simulink model "SIM_PEM_stack"  (R2020b)
settings: Solver=VariableStepAuto  StartTime=0.0  StopTime=60e3  RelTol=1e-3
undefined symbols (not defined in the file or in its folder): FC, FuelCellLoadFcn, gcbh, sps_rtmsupport
libraries: powerlib x106, simulink x22, spsFuelCellModel x21, dspswit3 x1, mylib x1
(part 2 of 3)

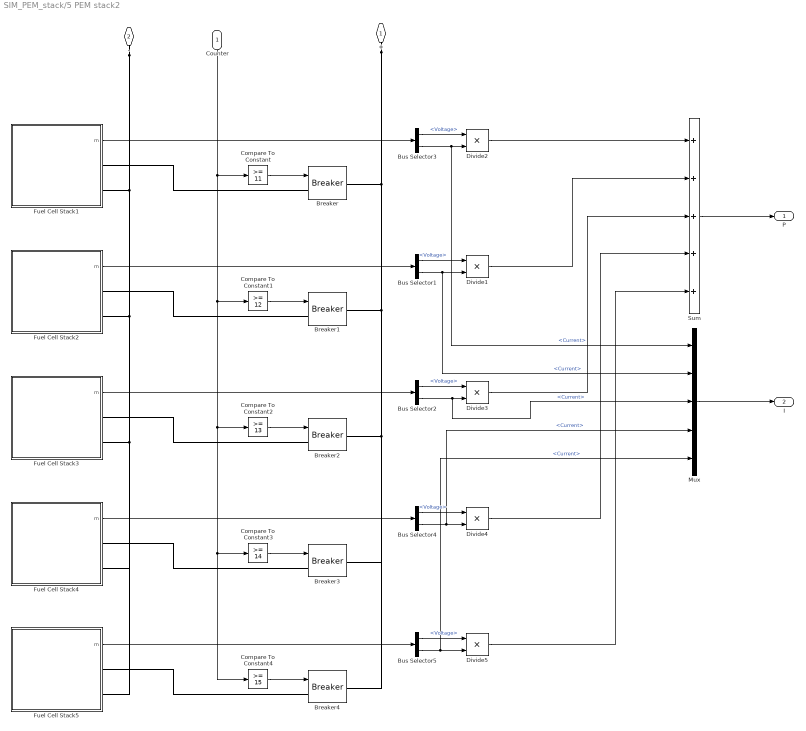
== system SIM_PEM_stack/5 PEM stack2 ==
  Counter : Inport
  Breaker{,1..4} (5 alike) : powerlib/Elements/Breaker  InitialState=0  SwitchingTimes="[1/60  5/60]"  External=on  BreakerResistance=0.01  SnubberResistance=1e6  SnubberCapacitance=inf  Measurements=None  MoreParameters=on  NoBreakLoop=off
  Bus Selector{1..5} (5 alike) : BusSelector  OutputSignals=Voltage,Current
  Compare To Constant : simulink/Logic and Bit Operations/Compare To Constant  relop=>=  const=11  OutDataTypeStr=boolean
  Compare To Constant1 : simulink/Logic and Bit Operations/Compare To Constant  relop=>=  const=12  OutDataTypeStr=boolean
  Compare To Constant2 : simulink/Logic and Bit Operations/Compare To Constant  relop=>=  const=13  OutDataTypeStr=boolean
  Compare To Constant3 : simulink/Logic and Bit Operations/Compare To Constant  relop=>=  const=14  OutDataTypeStr=boolean
  Compare To Constant4 : simulink/Logic and Bit Operations/Compare To Constant  relop=>=  const=15  OutDataTypeStr=boolean
  Divide{1..5} (5 alike) : Product  Inputs=**
  Fuel Cell Stack1 : Subsystem  AncestorBlock=electricdrivelib/Extra Sources/Fuel Cell Stack  DialogController=POWERSYS.PowerSysDialog  LoadFcn=sps_rtmsupport('LoadFcn',gcbh);FuelCellLoadFcn(gcb)  StartFcn=sps_rtmsupport('StartFcn',gcbh);  StopFcn=sps_rtmsupport('StopFcn',gcbh);  mask(Fuel Cell Stack){PresetModel=No (User-Defined), FcType=Proton Exchange Membrane (PEM), Detailed=Detailed, Eoc=[93.2,88], NomVI=[160,65.5], EndVI=[230,58.6], Nc=96, n=54, TOp=65, AirFr=510, SuppPress=[1.26,1], Comp=[99.95,21,1], SignX=off, SignY=off, FlowRateH2=off, FlowRateAir=off, SystemTemp=off, SystemPH2=off, SystemPAir=off, FCDyn=on, FC_tau=1, Peak_O2=80, V_Under=10}
      mask prompts: PresetModel "Preset model:"; FcType "Fuel Cell type:"; Detailed "Model detail Level:"; Eoc "Voltage at 0A and 1A [V_0(V), V_1(V)]"; NomVI "Nominal operating point [Inom(A), Vnom(V)]"; EndVI "Maximum operating point [Iend(A), Vend(V)]"; Nc "Number of cells"; n "Nominal stack efficiency (%)"; TOp "Operating temperature (Celsius)"; AirFr "Nominal Air flow rate (lpm)"; SuppPress "Nominal supply pressure [Fuel (bar), Air (bar)]"; Comp "Nominal composition (%) [H2 O2 H2O(Air)]"; SignX "Fuel  composition [x_H2(%)]"; SignY "Oxidant composition [y_O2(%)]"; FlowRateH2 "Fuel flow rate [FuelFr(lpm)]"; FlowRateAir "Air flow rate [AirFr(lpm)]"; SystemTemp "System Temperature [T(Kelvin)]"; SystemPH2 "Fuel supply pressure [Pfuel(bar)]"; SystemPAir "Air supply pressure [PAir(bar)]"; FCDyn "Specify Fuel Cell Dynamics?"; FC_tau "Fuel Cell response time (sec)"; Peak_O2 "Peak O2 utilization (%)"; V_Under "Voltage undershoot (V) @ peak O2 utilization"
      mask help:
      | Implements a generic hydrogen fuel cell model which allows the simulation for the following types of cells:
      | - Proton Exchange Membrane Fuel Cell (PEMFC)
      | - Solid Oxide Fuel Cell (SOFC)
      | - Alkaline Fuel Cell (AFC)
      mask init: same as SIM_PEM_stack/Fuel Cell Stack
      settings: CopyFcn=sps_rtmsupport('CopyFcn',gcbh);  DeleteFcn=sps_rtmsupport('DeleteFcn',gcbh);  UndoDeleteFcn=sps_rtmsupport('UndoDeleteFcn',gcbh);  ModelCloseFcn=sps_rtmsupport('ModelCloseFcn',gcbh);  PreSaveFcn=sps_rtmsupport('PreSaveFcn',gcbh);  PostSaveFcn=sps_rtmsupport('PostSaveFcn',gcbh);  NameChangeFcn=sps_rtmsupport('NameChangeFcn',gcbh);  PreCopyFcn=sps_rtmsupport('PreCopyFcn',gcbh);  OpenFcn=sps_rtmsupport('OpenFcn',gcbh, [1 2 3 13 14 15 16 17 18 19 20]);  CloseFcn=sps_rtmsupport('CloseFcn',gcbh);  PreDeleteFcn=sps_rtmsupport('PreDeleteFcn',gcbh);
      mask Help: helpview(psbhelp)
      mask TypeOptions PresetModel: No (User-Defined) | PEMFC - 1.26 kW - 24 Vdc | PEMFC - 6 kW - 45 Vdc | PEMFC - 50 kW - 625 Vdc | AFC - 2.4 kW - 48 Vdc | SOFC - 3 kW - 100 Vdc | SOFC - 25 kW - 630 Vdc
      mask Callback PresetModel: FuelCellCback(gcb,'Preset')
      mask TypeOptions Detailed: Simplified | Detailed
      mask Callback Detailed: FuelCellCback(gcb,'Visibilities')
      mask Callback FlowRateAir: FuelCellCback(gcb,'Visibilities')
      mask Callback FCDyn: FuelCellCback(gcb,'Visibilities')
      mask DialogControl ParameterTabVar0 Prompt: Parameters
      mask DialogControl plot_graph Prompt: Plot V_I characteristic
      mask DialogControl plot_graph Callback: FuelCellCback(gcb,'PlotGraph');
      mask DialogControl ViewParam Prompt: View Cell parameters
      mask DialogControl ViewParam Callback: FuelCellCback(gcb,'ViewParam');
      mask DialogControl ParameterTabVar01 Prompt: Signal variation
      mask DialogControl ParameterTabVar012 Prompt: Fuel Cell Dynamics
      mask Display: image(imread('power_fuelcell.png'));
  Fuel Cell Stack2 : Subsystem  AncestorBlock=electricdrivelib/Extra Sources/Fuel Cell Stack  DialogController=POWERSYS.PowerSysDialog  LoadFcn=sps_rtmsupport('LoadFcn',gcbh);FuelCellLoadFcn(gcb)  StartFcn=sps_rtmsupport('StartFcn',gcbh);  StopFcn=sps_rtmsupport('StopFcn',gcbh);  mask(Fuel Cell Stack){PresetModel=No (User-Defined), FcType=Proton Exchange Membrane (PEM), Detailed=Detailed, Eoc=[93.2,88], NomVI=[160,65.5], EndVI=[230,58.6], Nc=96, n=54, TOp=65, AirFr=510, SuppPress=[1.26,1], Comp=[99.95,21,1], SignX=off, SignY=off, FlowRateH2=off, FlowRateAir=off, SystemTemp=off, SystemPH2=off, SystemPAir=off, FCDyn=on, FC_tau=1, Peak_O2=80, V_Under=10}
      mask prompts: PresetModel "Preset model:"; FcType "Fuel Cell type:"; Detailed "Model detail Level:"; Eoc "Voltage at 0A and 1A [V_0(V), V_1(V)]"; NomVI "Nominal operating point [Inom(A), Vnom(V)]"; EndVI "Maximum operating point [Iend(A), Vend(V)]"; Nc "Number of cells"; n "Nominal stack efficiency (%)"; TOp "Operating temperature (Celsius)"; AirFr "Nominal Air flow rate (lpm)"; SuppPress "Nominal supply pressure [Fuel (bar), Air (bar)]"; Comp "Nominal composition (%) [H2 O2 H2O(Air)]"; SignX "Fuel  composition [x_H2(%)]"; SignY "Oxidant composition [y_O2(%)]"; FlowRateH2 "Fuel flow rate [FuelFr(lpm)]"; FlowRateAir "Air flow rate [AirFr(lpm)]"; SystemTemp "System Temperature [T(Kelvin)]"; SystemPH2 "Fuel supply pressure [Pfuel(bar)]"; SystemPAir "Air supply pressure [PAir(bar)]"; FCDyn "Specify Fuel Cell Dynamics?"; FC_tau "Fuel Cell response time (sec)"; Peak_O2 "Peak O2 utilization (%)"; V_Under "Voltage undershoot (V) @ peak O2 utilization"
      mask help:
      | Implements a generic hydrogen fuel cell model which allows the simulation for the following types of cells:
      | - Proton Exchange Membrane Fuel Cell (PEMFC)
      | - Solid Oxide Fuel Cell (SOFC)
      | - Alkaline Fuel Cell (AFC)
      mask init: same as SIM_PEM_stack/Fuel Cell Stack
      settings: CopyFcn=sps_rtmsupport('CopyFcn',gcbh);  DeleteFcn=sps_rtmsupport('DeleteFcn',gcbh);  UndoDeleteFcn=sps_rtmsupport('UndoDeleteFcn',gcbh);  ModelCloseFcn=sps_rtmsupport('ModelCloseFcn',gcbh);  PreSaveFcn=sps_rtmsupport('PreSaveFcn',gcbh);  PostSaveFcn=sps_rtmsupport('PostSaveFcn',gcbh);  NameChangeFcn=sps_rtmsupport('NameChangeFcn',gcbh);  PreCopyFcn=sps_rtmsupport('PreCopyFcn',gcbh);  OpenFcn=sps_rtmsupport('OpenFcn',gcbh, [1 2 3 13 14 15 16 17 18 19 20]);  CloseFcn=sps_rtmsupport('CloseFcn',gcbh);  PreDeleteFcn=sps_rtmsupport('PreDeleteFcn',gcbh);
      mask Help: helpview(psbhelp)
      mask TypeOptions PresetModel: No (User-Defined) | PEMFC - 1.26 kW - 24 Vdc | PEMFC - 6 kW - 45 Vdc | PEMFC - 50 kW - 625 Vdc | AFC - 2.4 kW - 48 Vdc | SOFC - 3 kW - 100 Vdc | SOFC - 25 kW - 630 Vdc
      mask Callback PresetModel: FuelCellCback(gcb,'Preset')
      mask TypeOptions Detailed: Simplified | Detailed
      mask Callback Detailed: FuelCellCback(gcb,'Visibilities')
      mask Callback FlowRateAir: FuelCellCback(gcb,'Visibilities')
      mask Callback FCDyn: FuelCellCback(gcb,'Visibilities')
      mask DialogControl ParameterTabVar0 Prompt: Parameters
      mask DialogControl plot_graph Prompt: Plot V_I characteristic
      mask DialogControl plot_graph Callback: FuelCellCback(gcb,'PlotGraph');
      mask DialogControl ViewParam Prompt: View Cell parameters
      mask DialogControl ViewParam Callback: FuelCellCback(gcb,'ViewParam');
      mask DialogControl ParameterTabVar01 Prompt: Signal variation
      mask DialogControl ParameterTabVar012 Prompt: Fuel Cell Dynamics
      mask Display: image(imread('power_fuelcell.png'));
  Fuel Cell Stack3 : Subsystem  AncestorBlock=electricdrivelib/Extra Sources/Fuel Cell Stack  DialogController=POWERSYS.PowerSysDialog  LoadFcn=sps_rtmsupport('LoadFcn',gcbh);FuelCellLoadFcn(gcb)  StartFcn=sps_rtmsupport('StartFcn',gcbh);  StopFcn=sps_rtmsupport('StopFcn',gcbh);  mask(Fuel Cell Stack){PresetModel=No (User-Defined), FcType=Proton Exchange Membrane (PEM), Detailed=Detailed, Eoc=[93.2,88], NomVI=[160,65.5], EndVI=[230,58.6], Nc=96, n=54, TOp=65, AirFr=510, SuppPress=[1.26,1], Comp=[99.95,21,1], SignX=off, SignY=off, FlowRateH2=off, FlowRateAir=off, SystemTemp=off, SystemPH2=off, SystemPAir=off, FCDyn=on, FC_tau=1, Peak_O2=80, V_Under=10}
      mask prompts: PresetModel "Preset model:"; FcType "Fuel Cell type:"; Detailed "Model detail Level:"; Eoc "Voltage at 0A and 1A [V_0(V), V_1(V)]"; NomVI "Nominal operating point [Inom(A), Vnom(V)]"; EndVI "Maximum operating point [Iend(A), Vend(V)]"; Nc "Number of cells"; n "Nominal stack efficiency (%)"; TOp "Operating temperature (Celsius)"; AirFr "Nominal Air flow rate (lpm)"; SuppPress "Nominal supply pressure [Fuel (bar), Air (bar)]"; Comp "Nominal composition (%) [H2 O2 H2O(Air)]"; SignX "Fuel  composition [x_H2(%)]"; SignY "Oxidant composition [y_O2(%)]"; FlowRateH2 "Fuel flow rate [FuelFr(lpm)]"; FlowRateAir "Air flow rate [AirFr(lpm)]"; SystemTemp "System Temperature [T(Kelvin)]"; SystemPH2 "Fuel supply pressure [Pfuel(bar)]"; SystemPAir "Air supply pressure [PAir(bar)]"; FCDyn "Specify Fuel Cell Dynamics?"; FC_tau "Fuel Cell response time (sec)"; Peak_O2 "Peak O2 utilization (%)"; V_Under "Voltage undershoot (V) @ peak O2 utilization"
      mask help:
      | Implements a generic hydrogen fuel cell model which allows the simulation for the following types of cells:
      | - Proton Exchange Membrane Fuel Cell (PEMFC)
      | - Solid Oxide Fuel Cell (SOFC)
      | - Alkaline Fuel Cell (AFC)
      mask init: same as SIM_PEM_stack/Fuel Cell Stack
      settings: CopyFcn=sps_rtmsupport('CopyFcn',gcbh);  DeleteFcn=sps_rtmsupport('DeleteFcn',gcbh);  UndoDeleteFcn=sps_rtmsupport('UndoDeleteFcn',gcbh);  ModelCloseFcn=sps_rtmsupport('ModelCloseFcn',gcbh);  PreSaveFcn=sps_rtmsupport('PreSaveFcn',gcbh);  PostSaveFcn=sps_rtmsupport('PostSaveFcn',gcbh);  NameChangeFcn=sps_rtmsupport('NameChangeFcn',gcbh);  PreCopyFcn=sps_rtmsupport('PreCopyFcn',gcbh);  OpenFcn=sps_rtmsupport('OpenFcn',gcbh, [1 2 3 13 14 15 16 17 18 19 20]);  CloseFcn=sps_rtmsupport('CloseFcn',gcbh);  PreDeleteFcn=sps_rtmsupport('PreDeleteFcn',gcbh);
      mask Help: helpview(psbhelp)
      mask TypeOptions PresetModel: No (User-Defined) | PEMFC - 1.26 kW - 24 Vdc | PEMFC - 6 kW - 45 Vdc | PEMFC - 50 kW - 625 Vdc | AFC - 2.4 kW - 48 Vdc | SOFC - 3 kW - 100 Vdc | SOFC - 25 kW - 630 Vdc
      mask Callback PresetModel: FuelCellCback(gcb,'Preset')
      mask TypeOptions Detailed: Simplified | Detailed
      mask Callback Detailed: FuelCellCback(gcb,'Visibilities')
      mask Callback FlowRateAir: FuelCellCback(gcb,'Visibilities')
      mask Callback FCDyn: FuelCellCback(gcb,'Visibilities')
      mask DialogControl ParameterTabVar0 Prompt: Parameters
      mask DialogControl plot_graph Prompt: Plot V_I characteristic
      mask DialogControl plot_graph Callback: FuelCellCback(gcb,'PlotGraph');
      mask DialogControl ViewParam Prompt: View Cell parameters
      mask DialogControl ViewParam Callback: FuelCellCback(gcb,'ViewParam');
      mask DialogControl ParameterTabVar01 Prompt: Signal variation
      mask DialogControl ParameterTabVar012 Prompt: Fuel Cell Dynamics
      mask Display: image(imread('power_fuelcell.png'));
  Fuel Cell Stack4 : Subsystem  AncestorBlock=electricdrivelib/Extra Sources/Fuel Cell Stack  DialogController=POWERSYS.PowerSysDialog  LoadFcn=sps_rtmsupport('LoadFcn',gcbh);FuelCellLoadFcn(gcb)  StartFcn=sps_rtmsupport('StartFcn',gcbh);  StopFcn=sps_rtmsupport('StopFcn',gcbh);  mask(Fuel Cell Stack){PresetModel=No (User-Defined), FcType=Proton Exchange Membrane (PEM), Detailed=Detailed, Eoc=[93.2,88], NomVI=[160,65.5], EndVI=[230,58.6], Nc=96, n=54, TOp=65, AirFr=510, SuppPress=[1.26,1], Comp=[99.95,21,1], SignX=off, SignY=off, FlowRateH2=off, FlowRateAir=off, SystemTemp=off, SystemPH2=off, SystemPAir=off, FCDyn=on, FC_tau=1, Peak_O2=80, V_Under=10}
      mask prompts: PresetModel "Preset model:"; FcType "Fuel Cell type:"; Detailed "Model detail Level:"; Eoc "Voltage at 0A and 1A [V_0(V), V_1(V)]"; NomVI "Nominal operating point [Inom(A), Vnom(V)]"; EndVI "Maximum operating point [Iend(A), Vend(V)]"; Nc "Number of cells"; n "Nominal stack efficiency (%)"; TOp "Operating temperature (Celsius)"; AirFr "Nominal Air flow rate (lpm)"; SuppPress "Nominal supply pressure [Fuel (bar), Air (bar)]"; Comp "Nominal composition (%) [H2 O2 H2O(Air)]"; SignX "Fuel  composition [x_H2(%)]"; SignY "Oxidant composition [y_O2(%)]"; FlowRateH2 "Fuel flow rate [FuelFr(lpm)]"; FlowRateAir "Air flow rate [AirFr(lpm)]"; SystemTemp "System Temperature [T(Kelvin)]"; SystemPH2 "Fuel supply pressure [Pfuel(bar)]"; SystemPAir "Air supply pressure [PAir(bar)]"; FCDyn "Specify Fuel Cell Dynamics?"; FC_tau "Fuel Cell response time (sec)"; Peak_O2 "Peak O2 utilization (%)"; V_Under "Voltage undershoot (V) @ peak O2 utilization"
      mask help:
      | Implements a generic hydrogen fuel cell model which allows the simulation for the following types of cells:
      | - Proton Exchange Membrane Fuel Cell (PEMFC)
      | - Solid Oxide Fuel Cell (SOFC)
      | - Alkaline Fuel Cell (AFC)
      mask init: same as SIM_PEM_stack/Fuel Cell Stack
      settings: CopyFcn=sps_rtmsupport('CopyFcn',gcbh);  DeleteFcn=sps_rtmsupport('DeleteFcn',gcbh);  UndoDeleteFcn=sps_rtmsupport('UndoDeleteFcn',gcbh);  ModelCloseFcn=sps_rtmsupport('ModelCloseFcn',gcbh);  PreSaveFcn=sps_rtmsupport('PreSaveFcn',gcbh);  PostSaveFcn=sps_rtmsupport('PostSaveFcn',gcbh);  NameChangeFcn=sps_rtmsupport('NameChangeFcn',gcbh);  PreCopyFcn=sps_rtmsupport('PreCopyFcn',gcbh);  OpenFcn=sps_rtmsupport('OpenFcn',gcbh, [1 2 3 13 14 15 16 17 18 19 20]);  CloseFcn=sps_rtmsupport('CloseFcn',gcbh);  PreDeleteFcn=sps_rtmsupport('PreDeleteFcn',gcbh);
      mask Help: helpview(psbhelp)
      mask TypeOptions PresetModel: No (User-Defined) | PEMFC - 1.26 kW - 24 Vdc | PEMFC - 6 kW - 45 Vdc | PEMFC - 50 kW - 625 Vdc | AFC - 2.4 kW - 48 Vdc | SOFC - 3 kW - 100 Vdc | SOFC - 25 kW - 630 Vdc
      mask Callback PresetModel: FuelCellCback(gcb,'Preset')
      mask TypeOptions Detailed: Simplified | Detailed
      mask Callback Detailed: FuelCellCback(gcb,'Visibilities')
      mask Callback FlowRateAir: FuelCellCback(gcb,'Visibilities')
      mask Callback FCDyn: FuelCellCback(gcb,'Visibilities')
      mask DialogControl ParameterTabVar0 Prompt: Parameters
      mask DialogControl plot_graph Prompt: Plot V_I characteristic
      mask DialogControl plot_graph Callback: FuelCellCback(gcb,'PlotGraph');
      mask DialogControl ViewParam Prompt: View Cell parameters
      mask DialogControl ViewParam Callback: FuelCellCback(gcb,'ViewParam');
      mask DialogControl ParameterTabVar01 Prompt: Signal variation
      mask DialogControl ParameterTabVar012 Prompt: Fuel Cell Dynamics
      mask Display: image(imread('power_fuelcell.png'));
  Fuel Cell Stack5 : Subsystem  AncestorBlock=electricdrivelib/Extra Sources/Fuel Cell Stack  DialogController=POWERSYS.PowerSysDialog  LoadFcn=sps_rtmsupport('LoadFcn',gcbh);FuelCellLoadFcn(gcb)  StartFcn=sps_rtmsupport('StartFcn',gcbh);  StopFcn=sps_rtmsupport('StopFcn',gcbh);  mask(Fuel Cell Stack){PresetModel=No (User-Defined), FcType=Proton Exchange Membrane (PEM), Detailed=Detailed, Eoc=[93.2,88], NomVI=[160,65.5], EndVI=[230,58.6], Nc=96, n=54, TOp=65, AirFr=510, SuppPress=[1.26,1], Comp=[99.95,21,1], SignX=off, SignY=off, FlowRateH2=off, FlowRateAir=off, SystemTemp=off, SystemPH2=off, SystemPAir=off, FCDyn=on, FC_tau=1, Peak_O2=80, V_Under=10}
      mask prompts: PresetModel "Preset model:"; FcType "Fuel Cell type:"; Detailed "Model detail Level:"; Eoc "Voltage at 0A and 1A [V_0(V), V_1(V)]"; NomVI "Nominal operating point [Inom(A), Vnom(V)]"; EndVI "Maximum operating point [Iend(A), Vend(V)]"; Nc "Number of cells"; n "Nominal stack efficiency (%)"; TOp "Operating temperature (Celsius)"; AirFr "Nominal Air flow rate (lpm)"; SuppPress "Nominal supply pressure [Fuel (bar), Air (bar)]"; Comp "Nominal composition (%) [H2 O2 H2O(Air)]"; SignX "Fuel  composition [x_H2(%)]"; SignY "Oxidant composition [y_O2(%)]"; FlowRateH2 "Fuel flow rate [FuelFr(lpm)]"; FlowRateAir "Air flow rate [AirFr(lpm)]"; SystemTemp "System Temperature [T(Kelvin)]"; SystemPH2 "Fuel supply pressure [Pfuel(bar)]"; SystemPAir "Air supply pressure [PAir(bar)]"; FCDyn "Specify Fuel Cell Dynamics?"; FC_tau "Fuel Cell response time (sec)"; Peak_O2 "Peak O2 utilization (%)"; V_Under "Voltage undershoot (V) @ peak O2 utilization"
      mask help:
      | Implements a generic hydrogen fuel cell model which allows the simulation for the following types of cells:
      | - Proton Exchange Membrane Fuel Cell (PEMFC)
      | - Solid Oxide Fuel Cell (SOFC)
      | - Alkaline Fuel Cell (AFC)
      mask init: same as SIM_PEM_stack/Fuel Cell Stack
      settings: CopyFcn=sps_rtmsupport('CopyFcn',gcbh);  DeleteFcn=sps_rtmsupport('DeleteFcn',gcbh);  UndoDeleteFcn=sps_rtmsupport('UndoDeleteFcn',gcbh);  ModelCloseFcn=sps_rtmsupport('ModelCloseFcn',gcbh);  PreSaveFcn=sps_rtmsupport('PreSaveFcn',gcbh);  PostSaveFcn=sps_rtmsupport('PostSaveFcn',gcbh);  NameChangeFcn=sps_rtmsupport('NameChangeFcn',gcbh);  PreCopyFcn=sps_rtmsupport('PreCopyFcn',gcbh);  OpenFcn=sps_rtmsupport('OpenFcn',gcbh, [1 2 3 13 14 15 16 17 18 19 20]);  CloseFcn=sps_rtmsupport('CloseFcn',gcbh);  PreDeleteFcn=sps_rtmsupport('PreDeleteFcn',gcbh);
      mask Help: helpview(psbhelp)
      mask TypeOptions PresetModel: No (User-Defined) | PEMFC - 1.26 kW - 24 Vdc | PEMFC - 6 kW - 45 Vdc | PEMFC - 50 kW - 625 Vdc | AFC - 2.4 kW - 48 Vdc | SOFC - 3 kW - 100 Vdc | SOFC - 25 kW - 630 Vdc
      mask Callback PresetModel: FuelCellCback(gcb,'Preset')
      mask TypeOptions Detailed: Simplified | Detailed
      mask Callback Detailed: FuelCellCback(gcb,'Visibilities')
      mask Callback FlowRateAir: FuelCellCback(gcb,'Visibilities')
      mask Callback FCDyn: FuelCellCback(gcb,'Visibilities')
      mask DialogControl ParameterTabVar0 Prompt: Parameters
      mask DialogControl plot_graph Prompt: Plot V_I characteristic
      mask DialogControl plot_graph Callback: FuelCellCback(gcb,'PlotGraph');
      mask DialogControl ViewParam Prompt: View Cell parameters
      mask DialogControl ViewParam Callback: FuelCellCback(gcb,'ViewParam');
      mask DialogControl ParameterTabVar01 Prompt: Signal variation
      mask DialogControl ParameterTabVar012 Prompt: Fuel Cell Dynamics
      mask Display: image(imread('power_fuelcell.png'));
  Mux : Mux  Inputs=5
  Sum : Sum  Inputs=+++++
  + : PMIOPort  Side=Left
  - : PMIOPort  Port=2  Side=Left
  P : Outport
  I : Outport  Port=2
  wires:
  Fuel Cell Stack1/1(m) -> Bus Selector3/1
  Bus Selector3/1 -> Divide2/1  "<Voltage>"
  Bus Selector3/2 -> Mux/1, Divide2/2  "<Current>"
  Compare To Constant/1 -> Breaker/1
  Bus Selector1/1 -> Divide1/1  "<Voltage>"
  Fuel Cell Stack2/1(m) -> Bus Selector1/1
  Bus Selector1/2 -> Mux/2, Divide1/2  "<Current>"
  Compare To Constant1/1 -> Breaker1/1
  Compare To Constant2/1 -> Breaker2/1
  Bus Selector2/2 -> Mux/3, Divide3/2  "<Current>"
  Bus Selector2/1 -> Divide3/1  "<Voltage>"
  Fuel Cell Stack3/1(m) -> Bus Selector2/1
  Compare To Constant3/1 -> Breaker3/1
  Bus Selector4/2 -> Mux/4, Divide4/2  "<Current>"
  Bus Selector4/1 -> Divide4/1  "<Voltage>"
  Fuel Cell Stack4/1(m) -> Bus Selector4/1
  Compare To Constant4/1 -> Breaker4/1
  Bus Selector5/2 -> Mux/5, Divide5/2  "<Current>"
  Bus Selector5/1 -> Divide5/1  "<Voltage>"
  Fuel Cell Stack5/1(m) -> Bus Selector5/1
  Counter/1 -> Compare To Constant4/1, Compare To Constant3/1, Compare To Constant2/1, Compare To Constant1/1, Compare To Constant/1
  Divide2/1 -> Sum/1
  Divide1/1 -> Sum/2
  Divide3/1 -> Sum/3
  Divide4/1 -> Sum/4
  Divide5/1 -> Sum/5
  Sum/1 -> P/1
  Mux/1 -> I/1
  connections:
  Breaker/LConn1 -- Fuel Cell Stack1/RConn1
  -/RConn1 -- Fuel Cell Stack1/RConn2 -- Fuel Cell Stack2/RConn2 -- Fuel Cell Stack3/RConn2 -- Fuel Cell Stack4/RConn2 -- Fuel Cell Stack5/RConn2
  +/RConn1 -- Breaker/RConn1 -- Breaker1/RConn1 -- Breaker2/RConn1 -- Breaker3/RConn1 -- Breaker4/RConn1
  Breaker1/LConn1 -- Fuel Cell Stack2/RConn1
  Breaker2/LConn1 -- Fuel Cell Stack3/RConn1
  Breaker3/LConn1 -- Fuel Cell Stack4/RConn1
  Breaker4/LConn1 -- Fuel Cell Stack5/RConn1

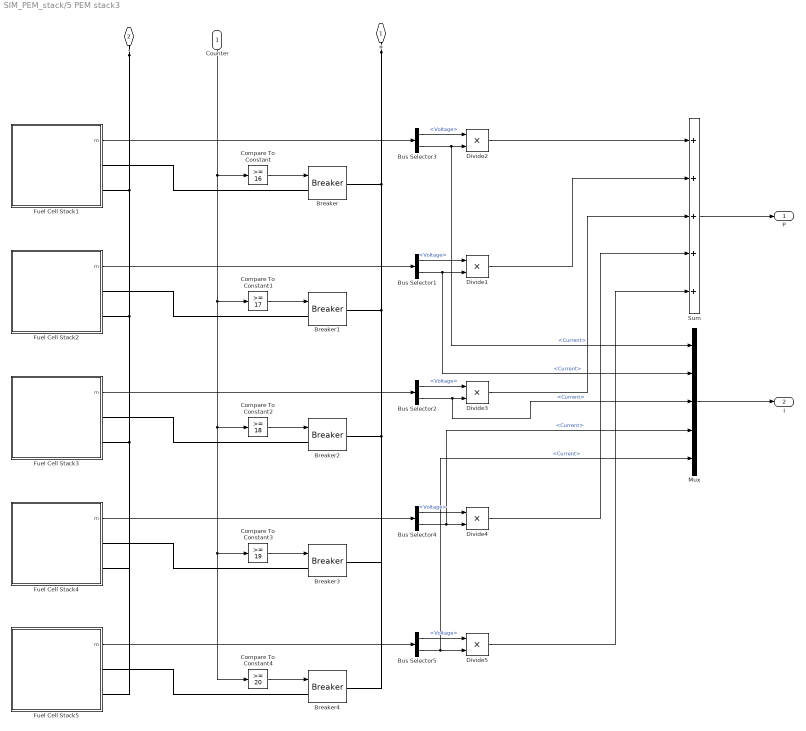
== system SIM_PEM_stack/5 PEM stack3 ==
  Counter : Inport
  Breaker{,1..4} (5 alike) : powerlib/Elements/Breaker  InitialState=0  SwitchingTimes="[1/60  5/60]"  External=on  BreakerResistance=0.01  SnubberResistance=1e6  SnubberCapacitance=inf  Measurements=None  MoreParameters=on  NoBreakLoop=off
  Bus Selector{1..5} (5 alike) : BusSelector  OutputSignals=Voltage,Current
  Compare To Constant : simulink/Logic and Bit Operations/Compare To Constant  relop=>=  const=16  OutDataTypeStr=boolean
  Compare To Constant1 : simulink/Logic and Bit Operations/Compare To Constant  relop=>=  const=17  OutDataTypeStr=boolean
  Compare To Constant2 : simulink/Logic and Bit Operations/Compare To Constant  relop=>=  const=18  OutDataTypeStr=boolean
  Compare To Constant3 : simulink/Logic and Bit Operations/Compare To Constant  relop=>=  const=19  OutDataTypeStr=boolean
  Compare To Constant4 : simulink/Logic and Bit Operations/Compare To Constant  relop=>=  const=20  OutDataTypeStr=boolean
  Divide{1..5} (5 alike) : Product  Inputs=**
  Fuel Cell Stack1 : Subsystem  AncestorBlock=electricdrivelib/Extra Sources/Fuel Cell Stack  DialogController=POWERSYS.PowerSysDialog  LoadFcn=sps_rtmsupport('LoadFcn',gcbh);FuelCellLoadFcn(gcb)  StartFcn=sps_rtmsupport('StartFcn',gcbh);  StopFcn=sps_rtmsupport('StopFcn',gcbh);  mask(Fuel Cell Stack){PresetModel=No (User-Defined), FcType=Proton Exchange Membrane (PEM), Detailed=Detailed, Eoc=[93.2,88], NomVI=[160,65.5], EndVI=[230,58.6], Nc=96, n=54, TOp=65, AirFr=510, SuppPress=[1.26,1], Comp=[99.95,21,1], SignX=off, SignY=off, FlowRateH2=off, FlowRateAir=off, SystemTemp=off, SystemPH2=off, SystemPAir=off, FCDyn=on, FC_tau=1, Peak_O2=80, V_Under=10}
      mask prompts: PresetModel "Preset model:"; FcType "Fuel Cell type:"; Detailed "Model detail Level:"; Eoc "Voltage at 0A and 1A [V_0(V), V_1(V)]"; NomVI "Nominal operating point [Inom(A), Vnom(V)]"; EndVI "Maximum operating point [Iend(A), Vend(V)]"; Nc "Number of cells"; n "Nominal stack efficiency (%)"; TOp "Operating temperature (Celsius)"; AirFr "Nominal Air flow rate (lpm)"; SuppPress "Nominal supply pressure [Fuel (bar), Air (bar)]"; Comp "Nominal composition (%) [H2 O2 H2O(Air)]"; SignX "Fuel  composition [x_H2(%)]"; SignY "Oxidant composition [y_O2(%)]"; FlowRateH2 "Fuel flow rate [FuelFr(lpm)]"; FlowRateAir "Air flow rate [AirFr(lpm)]"; SystemTemp "System Temperature [T(Kelvin)]"; SystemPH2 "Fuel supply pressure [Pfuel(bar)]"; SystemPAir "Air supply pressure [PAir(bar)]"; FCDyn "Specify Fuel Cell Dynamics?"; FC_tau "Fuel Cell response time (sec)"; Peak_O2 "Peak O2 utilization (%)"; V_Under "Voltage undershoot (V) @ peak O2 utilization"
      mask help:
      | Implements a generic hydrogen fuel cell model which allows the simulation for the following types of cells:
      | - Proton Exchange Membrane Fuel Cell (PEMFC)
      | - Solid Oxide Fuel Cell (SOFC)
      | - Alkaline Fuel Cell (AFC)
      mask init: same as SIM_PEM_stack/Fuel Cell Stack
      settings: CopyFcn=sps_rtmsupport('CopyFcn',gcbh);  DeleteFcn=sps_rtmsupport('DeleteFcn',gcbh);  UndoDeleteFcn=sps_rtmsupport('UndoDeleteFcn',gcbh);  ModelCloseFcn=sps_rtmsupport('ModelCloseFcn',gcbh);  PreSaveFcn=sps_rtmsupport('PreSaveFcn',gcbh);  PostSaveFcn=sps_rtmsupport('PostSaveFcn',gcbh);  NameChangeFcn=sps_rtmsupport('NameChangeFcn',gcbh);  PreCopyFcn=sps_rtmsupport('PreCopyFcn',gcbh);  OpenFcn=sps_rtmsupport('OpenFcn',gcbh, [1 2 3 13 14 15 16 17 18 19 20]);  CloseFcn=sps_rtmsupport('CloseFcn',gcbh);  PreDeleteFcn=sps_rtmsupport('PreDeleteFcn',gcbh);
      mask Help: helpview(psbhelp)
      mask TypeOptions PresetModel: No (User-Defined) | PEMFC - 1.26 kW - 24 Vdc | PEMFC - 6 kW - 45 Vdc | PEMFC - 50 kW - 625 Vdc | AFC - 2.4 kW - 48 Vdc | SOFC - 3 kW - 100 Vdc | SOFC - 25 kW - 630 Vdc
      mask Callback PresetModel: FuelCellCback(gcb,'Preset')
      mask TypeOptions Detailed: Simplified | Detailed
      mask Callback Detailed: FuelCellCback(gcb,'Visibilities')
      mask Callback FlowRateAir: FuelCellCback(gcb,'Visibilities')
      mask Callback FCDyn: FuelCellCback(gcb,'Visibilities')
      mask DialogControl ParameterTabVar0 Prompt: Parameters
      mask DialogControl plot_graph Prompt: Plot V_I characteristic
      mask DialogControl plot_graph Callback: FuelCellCback(gcb,'PlotGraph');
      mask DialogControl ViewParam Prompt: View Cell parameters
      mask DialogControl ViewParam Callback: FuelCellCback(gcb,'ViewParam');
      mask DialogControl ParameterTabVar01 Prompt: Signal variation
      mask DialogControl ParameterTabVar012 Prompt: Fuel Cell Dynamics
      mask Display: image(imread('power_fuelcell.png'));
  Fuel Cell Stack2 : Subsystem  AncestorBlock=electricdrivelib/Extra Sources/Fuel Cell Stack  DialogController=POWERSYS.PowerSysDialog  LoadFcn=sps_rtmsupport('LoadFcn',gcbh);FuelCellLoadFcn(gcb)  StartFcn=sps_rtmsupport('StartFcn',gcbh);  StopFcn=sps_rtmsupport('StopFcn',gcbh);  mask(Fuel Cell Stack){PresetModel=No (User-Defined), FcType=Proton Exchange Membrane (PEM), Detailed=Detailed, Eoc=[93.2,88], NomVI=[160,65.5], EndVI=[230,58.6], Nc=96, n=54, TOp=65, AirFr=510, SuppPress=[1.26,1], Comp=[99.95,21,1], SignX=off, SignY=off, FlowRateH2=off, FlowRateAir=off, SystemTemp=off, SystemPH2=off, SystemPAir=off, FCDyn=on, FC_tau=1, Peak_O2=80, V_Under=10}
      mask prompts: PresetModel "Preset model:"; FcType "Fuel Cell type:"; Detailed "Model detail Level:"; Eoc "Voltage at 0A and 1A [V_0(V), V_1(V)]"; NomVI "Nominal operating point [Inom(A), Vnom(V)]"; EndVI "Maximum operating point [Iend(A), Vend(V)]"; Nc "Number of cells"; n "Nominal stack efficiency (%)"; TOp "Operating temperature (Celsius)"; AirFr "Nominal Air flow rate (lpm)"; SuppPress "Nominal supply pressure [Fuel (bar), Air (bar)]"; Comp "Nominal composition (%) [H2 O2 H2O(Air)]"; SignX "Fuel  composition [x_H2(%)]"; SignY "Oxidant composition [y_O2(%)]"; FlowRateH2 "Fuel flow rate [FuelFr(lpm)]"; FlowRateAir "Air flow rate [AirFr(lpm)]"; SystemTemp "System Temperature [T(Kelvin)]"; SystemPH2 "Fuel supply pressure [Pfuel(bar)]"; SystemPAir "Air supply pressure [PAir(bar)]"; FCDyn "Specify Fuel Cell Dynamics?"; FC_tau "Fuel Cell response time (sec)"; Peak_O2 "Peak O2 utilization (%)"; V_Under "Voltage undershoot (V) @ peak O2 utilization"
      mask help:
      | Implements a generic hydrogen fuel cell model which allows the simulation for the following types of cells:
      | - Proton Exchange Membrane Fuel Cell (PEMFC)
      | - Solid Oxide Fuel Cell (SOFC)
      | - Alkaline Fuel Cell (AFC)
      mask init: same as SIM_PEM_stack/Fuel Cell Stack
      settings: CopyFcn=sps_rtmsupport('CopyFcn',gcbh);  DeleteFcn=sps_rtmsupport('DeleteFcn',gcbh);  UndoDeleteFcn=sps_rtmsupport('UndoDeleteFcn',gcbh);  ModelCloseFcn=sps_rtmsupport('ModelCloseFcn',gcbh);  PreSaveFcn=sps_rtmsupport('PreSaveFcn',gcbh);  PostSaveFcn=sps_rtmsupport('PostSaveFcn',gcbh);  NameChangeFcn=sps_rtmsupport('NameChangeFcn',gcbh);  PreCopyFcn=sps_rtmsupport('PreCopyFcn',gcbh);  OpenFcn=sps_rtmsupport('OpenFcn',gcbh, [1 2 3 13 14 15 16 17 18 19 20]);  CloseFcn=sps_rtmsupport('CloseFcn',gcbh);  PreDeleteFcn=sps_rtmsupport('PreDeleteFcn',gcbh);
      mask Help: helpview(psbhelp)
      mask TypeOptions PresetModel: No (User-Defined) | PEMFC - 1.26 kW - 24 Vdc | PEMFC - 6 kW - 45 Vdc | PEMFC - 50 kW - 625 Vdc | AFC - 2.4 kW - 48 Vdc | SOFC - 3 kW - 100 Vdc | SOFC - 25 kW - 630 Vdc
      mask Callback PresetModel: FuelCellCback(gcb,'Preset')
      mask TypeOptions Detailed: Simplified | Detailed
      mask Callback Detailed: FuelCellCback(gcb,'Visibilities')
      mask Callback FlowRateAir: FuelCellCback(gcb,'Visibilities')
      mask Callback FCDyn: FuelCellCback(gcb,'Visibilities')
      mask DialogControl ParameterTabVar0 Prompt: Parameters
      mask DialogControl plot_graph Prompt: Plot V_I characteristic
      mask DialogControl plot_graph Callback: FuelCellCback(gcb,'PlotGraph');
      mask DialogControl ViewParam Prompt: View Cell parameters
      mask DialogControl ViewParam Callback: FuelCellCback(gcb,'ViewParam');
      mask DialogControl ParameterTabVar01 Prompt: Signal variation
      mask DialogControl ParameterTabVar012 Prompt: Fuel Cell Dynamics
      mask Display: image(imread('power_fuelcell.png'));
  Fuel Cell Stack3 : Subsystem  AncestorBlock=electricdrivelib/Extra Sources/Fuel Cell Stack  DialogController=POWERSYS.PowerSysDialog  LoadFcn=sps_rtmsupport('LoadFcn',gcbh);FuelCellLoadFcn(gcb)  StartFcn=sps_rtmsupport('StartFcn',gcbh);  StopFcn=sps_rtmsupport('StopFcn',gcbh);  mask(Fuel Cell Stack){PresetModel=No (User-Defined), FcType=Proton Exchange Membrane (PEM), Detailed=Detailed, Eoc=[93.2,88], NomVI=[160,65.5], EndVI=[230,58.6], Nc=96, n=54, TOp=65, AirFr=510, SuppPress=[1.26,1], Comp=[99.95,21,1], SignX=off, SignY=off, FlowRateH2=off, FlowRateAir=off, SystemTemp=off, SystemPH2=off, SystemPAir=off, FCDyn=on, FC_tau=1, Peak_O2=80, V_Under=10}
      mask prompts: PresetModel "Preset model:"; FcType "Fuel Cell type:"; Detailed "Model detail Level:"; Eoc "Voltage at 0A and 1A [V_0(V), V_1(V)]"; NomVI "Nominal operating point [Inom(A), Vnom(V)]"; EndVI "Maximum operating point [Iend(A), Vend(V)]"; Nc "Number of cells"; n "Nominal stack efficiency (%)"; TOp "Operating temperature (Celsius)"; AirFr "Nominal Air flow rate (lpm)"; SuppPress "Nominal supply pressure [Fuel (bar), Air (bar)]"; Comp "Nominal composition (%) [H2 O2 H2O(Air)]"; SignX "Fuel  composition [x_H2(%)]"; SignY "Oxidant composition [y_O2(%)]"; FlowRateH2 "Fuel flow rate [FuelFr(lpm)]"; FlowRateAir "Air flow rate [AirFr(lpm)]"; SystemTemp "System Temperature [T(Kelvin)]"; SystemPH2 "Fuel supply pressure [Pfuel(bar)]"; SystemPAir "Air supply pressure [PAir(bar)]"; FCDyn "Specify Fuel Cell Dynamics?"; FC_tau "Fuel Cell response time (sec)"; Peak_O2 "Peak O2 utilization (%)"; V_Under "Voltage undershoot (V) @ peak O2 utilization"
      mask help:
      | Implements a generic hydrogen fuel cell model which allows the simulation for the following types of cells:
      | - Proton Exchange Membrane Fuel Cell (PEMFC)
      | - Solid Oxide Fuel Cell (SOFC)
      | - Alkaline Fuel Cell (AFC)
      mask init: same as SIM_PEM_stack/Fuel Cell Stack
      settings: CopyFcn=sps_rtmsupport('CopyFcn',gcbh);  DeleteFcn=sps_rtmsupport('DeleteFcn',gcbh);  UndoDeleteFcn=sps_rtmsupport('UndoDeleteFcn',gcbh);  ModelCloseFcn=sps_rtmsupport('ModelCloseFcn',gcbh);  PreSaveFcn=sps_rtmsupport('PreSaveFcn',gcbh);  PostSaveFcn=sps_rtmsupport('PostSaveFcn',gcbh);  NameChangeFcn=sps_rtmsupport('NameChangeFcn',gcbh);  PreCopyFcn=sps_rtmsupport('PreCopyFcn',gcbh);  OpenFcn=sps_rtmsupport('OpenFcn',gcbh, [1 2 3 13 14 15 16 17 18 19 20]);  CloseFcn=sps_rtmsupport('CloseFcn',gcbh);  PreDeleteFcn=sps_rtmsupport('PreDeleteFcn',gcbh);
      mask Help: helpview(psbhelp)
      mask TypeOptions PresetModel: No (User-Defined) | PEMFC - 1.26 kW - 24 Vdc | PEMFC - 6 kW - 45 Vdc | PEMFC - 50 kW - 625 Vdc | AFC - 2.4 kW - 48 Vdc | SOFC - 3 kW - 100 Vdc | SOFC - 25 kW - 630 Vdc
      mask Callback PresetModel: FuelCellCback(gcb,'Preset')
      mask TypeOptions Detailed: Simplified | Detailed
      mask Callback Detailed: FuelCellCback(gcb,'Visibilities')
      mask Callback FlowRateAir: FuelCellCback(gcb,'Visibilities')
      mask Callback FCDyn: FuelCellCback(gcb,'Visibilities')
      mask DialogControl ParameterTabVar0 Prompt: Parameters
      mask DialogControl plot_graph Prompt: Plot V_I characteristic
      mask DialogControl plot_graph Callback: FuelCellCback(gcb,'PlotGraph');
      mask DialogControl ViewParam Prompt: View Cell parameters
      mask DialogControl ViewParam Callback: FuelCellCback(gcb,'ViewParam');
      mask DialogControl ParameterTabVar01 Prompt: Signal variation
      mask DialogControl ParameterTabVar012 Prompt: Fuel Cell Dynamics
      mask Display: image(imread('power_fuelcell.png'));
  Fuel Cell Stack4 : Subsystem  AncestorBlock=electricdrivelib/Extra Sources/Fuel Cell Stack  DialogController=POWERSYS.PowerSysDialog  LoadFcn=sps_rtmsupport('LoadFcn',gcbh);FuelCellLoadFcn(gcb)  StartFcn=sps_rtmsupport('StartFcn',gcbh);  StopFcn=sps_rtmsupport('StopFcn',gcbh);  mask(Fuel Cell Stack){PresetModel=No (User-Defined), FcType=Proton Exchange Membrane (PEM), Detailed=Detailed, Eoc=[93.2,88], NomVI=[160,65.5], EndVI=[230,58.6], Nc=96, n=54, TOp=65, AirFr=510, SuppPress=[1.26,1], Comp=[99.95,21,1], SignX=off, SignY=off, FlowRateH2=off, FlowRateAir=off, SystemTemp=off, SystemPH2=off, SystemPAir=off, FCDyn=on, FC_tau=1, Peak_O2=80, V_Under=10}
      mask prompts: PresetModel "Preset model:"; FcType "Fuel Cell type:"; Detailed "Model detail Level:"; Eoc "Voltage at 0A and 1A [V_0(V), V_1(V)]"; NomVI "Nominal operating point [Inom(A), Vnom(V)]"; EndVI "Maximum operating point [Iend(A), Vend(V)]"; Nc "Number of cells"; n "Nominal stack efficiency (%)"; TOp "Operating temperature (Celsius)"; AirFr "Nominal Air flow rate (lpm)"; SuppPress "Nominal supply pressure [Fuel (bar), Air (bar)]"; Comp "Nominal composition (%) [H2 O2 H2O(Air)]"; SignX "Fuel  composition [x_H2(%)]"; SignY "Oxidant composition [y_O2(%)]"; FlowRateH2 "Fuel flow rate [FuelFr(lpm)]"; FlowRateAir "Air flow rate [AirFr(lpm)]"; SystemTemp "System Temperature [T(Kelvin)]"; SystemPH2 "Fuel supply pressure [Pfuel(bar)]"; SystemPAir "Air supply pressure [PAir(bar)]"; FCDyn "Specify Fuel Cell Dynamics?"; FC_tau "Fuel Cell response time (sec)"; Peak_O2 "Peak O2 utilization (%)"; V_Under "Voltage undershoot (V) @ peak O2 utilization"
      mask help:
      | Implements a generic hydrogen fuel cell model which allows the simulation for the following types of cells:
      | - Proton Exchange Membrane Fuel Cell (PEMFC)
      | - Solid Oxide Fuel Cell (SOFC)
      | - Alkaline Fuel Cell (AFC)
      mask init: same as SIM_PEM_stack/Fuel Cell Stack
      settings: CopyFcn=sps_rtmsupport('CopyFcn',gcbh);  DeleteFcn=sps_rtmsupport('DeleteFcn',gcbh);  UndoDeleteFcn=sps_rtmsupport('UndoDeleteFcn',gcbh);  ModelCloseFcn=sps_rtmsupport('ModelCloseFcn',gcbh);  PreSaveFcn=sps_rtmsupport('PreSaveFcn',gcbh);  PostSaveFcn=sps_rtmsupport('PostSaveFcn',gcbh);  NameChangeFcn=sps_rtmsupport('NameChangeFcn',gcbh);  PreCopyFcn=sps_rtmsupport('PreCopyFcn',gcbh);  OpenFcn=sps_rtmsupport('OpenFcn',gcbh, [1 2 3 13 14 15 16 17 18 19 20]);  CloseFcn=sps_rtmsupport('CloseFcn',gcbh);  PreDeleteFcn=sps_rtmsupport('PreDeleteFcn',gcbh);
      mask Help: helpview(psbhelp)
      mask TypeOptions PresetModel: No (User-Defined) | PEMFC - 1.26 kW - 24 Vdc | PEMFC - 6 kW - 45 Vdc | PEMFC - 50 kW - 625 Vdc | AFC - 2.4 kW - 48 Vdc | SOFC - 3 kW - 100 Vdc | SOFC - 25 kW - 630 Vdc
      mask Callback PresetModel: FuelCellCback(gcb,'Preset')
      mask TypeOptions Detailed: Simplified | Detailed
      mask Callback Detailed: FuelCellCback(gcb,'Visibilities')
      mask Callback FlowRateAir: FuelCellCback(gcb,'Visibilities')
      mask Callback FCDyn: FuelCellCback(gcb,'Visibilities')
      mask DialogControl ParameterTabVar0 Prompt: Parameters
      mask DialogControl plot_graph Prompt: Plot V_I characteristic
      mask DialogControl plot_graph Callback: FuelCellCback(gcb,'PlotGraph');
      mask DialogControl ViewParam Prompt: View Cell parameters
      mask DialogControl ViewParam Callback: FuelCellCback(gcb,'ViewParam');
      mask DialogControl ParameterTabVar01 Prompt: Signal variation
      mask DialogControl ParameterTabVar012 Prompt: Fuel Cell Dynamics
      mask Display: image(imread('power_fuelcell.png'));
  Fuel Cell Stack5 : Subsystem  AncestorBlock=electricdrivelib/Extra Sources/Fuel Cell Stack  DialogController=POWERSYS.PowerSysDialog  LoadFcn=sps_rtmsupport('LoadFcn',gcbh);FuelCellLoadFcn(gcb)  StartFcn=sps_rtmsupport('StartFcn',gcbh);  StopFcn=sps_rtmsupport('StopFcn',gcbh);  mask(Fuel Cell Stack){PresetModel=No (User-Defined), FcType=Proton Exchange Membrane (PEM), Detailed=Detailed, Eoc=[93.2,88], NomVI=[160,65.5], EndVI=[230,58.6], Nc=96, n=54, TOp=65, AirFr=510, SuppPress=[1.26,1], Comp=[99.95,21,1], SignX=off, SignY=off, FlowRateH2=off, FlowRateAir=off, SystemTemp=off, SystemPH2=off, SystemPAir=off, FCDyn=on, FC_tau=1, Peak_O2=80, V_Under=10}
      mask prompts: PresetModel "Preset model:"; FcType "Fuel Cell type:"; Detailed "Model detail Level:"; Eoc "Voltage at 0A and 1A [V_0(V), V_1(V)]"; NomVI "Nominal operating point [Inom(A), Vnom(V)]"; EndVI "Maximum operating point [Iend(A), Vend(V)]"; Nc "Number of cells"; n "Nominal stack efficiency (%)"; TOp "Operating temperature (Celsius)"; AirFr "Nominal Air flow rate (lpm)"; SuppPress "Nominal supply pressure [Fuel (bar), Air (bar)]"; Comp "Nominal composition (%) [H2 O2 H2O(Air)]"; SignX "Fuel  composition [x_H2(%)]"; SignY "Oxidant composition [y_O2(%)]"; FlowRateH2 "Fuel flow rate [FuelFr(lpm)]"; FlowRateAir "Air flow rate [AirFr(lpm)]"; SystemTemp "System Temperature [T(Kelvin)]"; SystemPH2 "Fuel supply pressure [Pfuel(bar)]"; SystemPAir "Air supply pressure [PAir(bar)]"; FCDyn "Specify Fuel Cell Dynamics?"; FC_tau "Fuel Cell response time (sec)"; Peak_O2 "Peak O2 utilization (%)"; V_Under "Voltage undershoot (V) @ peak O2 utilization"
      mask help:
      | Implements a generic hydrogen fuel cell model which allows the simulation for the following types of cells:
      | - Proton Exchange Membrane Fuel Cell (PEMFC)
      | - Solid Oxide Fuel Cell (SOFC)
      | - Alkaline Fuel Cell (AFC)
      mask init: same as SIM_PEM_stack/Fuel Cell Stack
      settings: CopyFcn=sps_rtmsupport('CopyFcn',gcbh);  DeleteFcn=sps_rtmsupport('DeleteFcn',gcbh);  UndoDeleteFcn=sps_rtmsupport('UndoDeleteFcn',gcbh);  ModelCloseFcn=sps_rtmsupport('ModelCloseFcn',gcbh);  PreSaveFcn=sps_rtmsupport('PreSaveFcn',gcbh);  PostSaveFcn=sps_rtmsupport('PostSaveFcn',gcbh);  NameChangeFcn=sps_rtmsupport('NameChangeFcn',gcbh);  PreCopyFcn=sps_rtmsupport('PreCopyFcn',gcbh);  OpenFcn=sps_rtmsupport('OpenFcn',gcbh, [1 2 3 13 14 15 16 17 18 19 20]);  CloseFcn=sps_rtmsupport('CloseFcn',gcbh);  PreDeleteFcn=sps_rtmsupport('PreDeleteFcn',gcbh);
      mask Help: helpview(psbhelp)
      mask TypeOptions PresetModel: No (User-Defined) | PEMFC - 1.26 kW - 24 Vdc | PEMFC - 6 kW - 45 Vdc | PEMFC - 50 kW - 625 Vdc | AFC - 2.4 kW - 48 Vdc | SOFC - 3 kW - 100 Vdc | SOFC - 25 kW - 630 Vdc
      mask Callback PresetModel: FuelCellCback(gcb,'Preset')
      mask TypeOptions Detailed: Simplified | Detailed
      mask Callback Detailed: FuelCellCback(gcb,'Visibilities')
      mask Callback FlowRateAir: FuelCellCback(gcb,'Visibilities')
      mask Callback FCDyn: FuelCellCback(gcb,'Visibilities')
      mask DialogControl ParameterTabVar0 Prompt: Parameters
      mask DialogControl plot_graph Prompt: Plot V_I characteristic
      mask DialogControl plot_graph Callback: FuelCellCback(gcb,'PlotGraph');
      mask DialogControl ViewParam Prompt: View Cell parameters
      mask DialogControl ViewParam Callback: FuelCellCback(gcb,'ViewParam');
      mask DialogControl ParameterTabVar01 Prompt: Signal variation
      mask DialogControl ParameterTabVar012 Prompt: Fuel Cell Dynamics
      mask Display: image(imread('power_fuelcell.png'));
  Mux : Mux  Inputs=5
  Sum : Sum  Inputs=+++++
  + : PMIOPort  Side=Left
  - : PMIOPort  Port=2  Side=Left
  P : Outport
  I : Outport  Port=2
  wires:
  Fuel Cell Stack1/1(m) -> Bus Selector3/1
  Bus Selector3/1 -> Divide2/1  "<Voltage>"
  Bus Selector3/2 -> Mux/1, Divide2/2  "<Current>"
  Compare To Constant/1 -> Breaker/1
  Bus Selector1/1 -> Divide1/1  "<Voltage>"
  Fuel Cell Stack2/1(m) -> Bus Selector1/1
  Bus Selector1/2 -> Mux/2, Divide1/2  "<Current>"
  Compare To Constant1/1 -> Breaker1/1
  Compare To Constant2/1 -> Breaker2/1
  Bus Selector2/2 -> Mux/3, Divide3/2  "<Current>"
  Bus Selector2/1 -> Divide3/1  "<Voltage>"
  Fuel Cell Stack3/1(m) -> Bus Selector2/1
  Compare To Constant3/1 -> Breaker3/1
  Bus Selector4/2 -> Mux/4, Divide4/2  "<Current>"
  Bus Selector4/1 -> Divide4/1  "<Voltage>"
  Fuel Cell Stack4/1(m) -> Bus Selector4/1
  Compare To Constant4/1 -> Breaker4/1
  Bus Selector5/2 -> Mux/5, Divide5/2  "<Current>"
  Bus Selector5/1 -> Divide5/1  "<Voltage>"
  Fuel Cell Stack5/1(m) -> Bus Selector5/1
  Counter/1 -> Compare To Constant4/1, Compare To Constant3/1, Compare To Constant2/1, Compare To Constant1/1, Compare To Constant/1
  Divide2/1 -> Sum/1
  Divide1/1 -> Sum/2
  Divide3/1 -> Sum/3
  Divide4/1 -> Sum/4
  Divide5/1 -> Sum/5
  Sum/1 -> P/1
  Mux/1 -> I/1
  connections:
  Breaker/LConn1 -- Fuel Cell Stack1/RConn1
  -/RConn1 -- Fuel Cell Stack1/RConn2 -- Fuel Cell Stack2/RConn2 -- Fuel Cell Stack3/RConn2 -- Fuel Cell Stack4/RConn2 -- Fuel Cell Stack5/RConn2
  +/RConn1 -- Breaker/RConn1 -- Breaker1/RConn1 -- Breaker2/RConn1 -- Breaker3/RConn1 -- Breaker4/RConn1
  Breaker1/LConn1 -- Fuel Cell Stack2/RConn1
  Breaker2/LConn1 -- Fuel Cell Stack3/RConn1
  Breaker3/LConn1 -- Fuel Cell Stack4/RConn1
  Breaker4/LConn1 -- Fuel Cell Stack5/RConn1

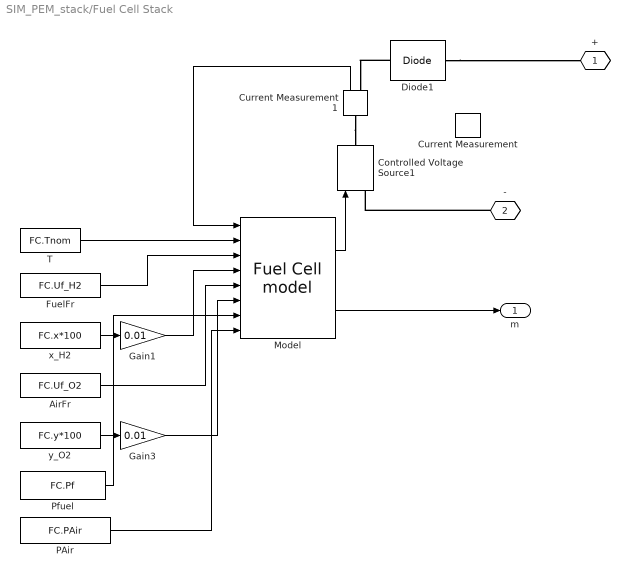
== system SIM_PEM_stack/Fuel Cell Stack ==
  AirFr : Constant  Value=FC.Uf_O2
  Controlled Voltage Source1 : powerlib/Electrical Sources/Controlled Voltage Source  Initialize=on  Source_Type=AC  Amplitude=0  Phase=0  Frequency=0  Measurements=None
  Current Measurement : powerlib/Measurements/Current Measurement  PhasorSimulation=off  OutputType=Complex  PSBequivalent=0
  Current Measurement1 : powerlib/Measurements/Current Measurement  PhasorSimulation=off  OutputType=Complex  PSBequivalent=0
  Diode1 : powerlib/Power Electronics/Diode  Ron=FC.Rohm  Lon=0  Vf=0  IC=0  UseSnubber=off  Rs=1e4  Cs=inf  Measurements=off
  FuelFr : Constant  Value=FC.Uf_H2
  Gain1 : Gain  Gain=0.01
  Gain3 : Gain  Gain=0.01
  Model : spsFuelCellModel/Fuel Cell model  SystemSampleTime=-1  LabelModeActiveChoice=Continuous/Detailed  VariantActivationTime=update diagram  Latency=0  AutoFrameSizeCalculation=off
      settings: AttributesFormatString=%<BlockChoice>  SourceProductBaseCode=PS
  PAir : Constant  Value=FC.PAir
  Pfuel : Constant  Value=FC.Pf
  T : Constant  Value=FC.Tnom
  x_H2 : Constant  Value=FC.x*100
  y_O2 : Constant  Value=FC.y*100
  + : PMIOPort  Tag=PMCPort  Side=Right
  - : PMIOPort  Tag=PMCPort  Port=2  Side=Right
  m : Outport  VectorParamsAs1DForOutWhenUnconnected=off
  wires:
  PAir/1 -> Model/8
  Pfuel/1 -> Model/7
  T/1 -> Model/2
  Model/1 -> Controlled Voltage Source1/1
  Current Measurement1/1 -> Model/1
  Model/2 -> m/1
  FuelFr/1 -> Model/3
  x_H2/1 -> Gain1/1
  AirFr/1 -> Model/5
  y_O2/1 -> Gain3/1
  Gain1/1 -> Model/4
  Gain3/1 -> Model/6
  connections:
  Current Measurement1/LConn1 -- Controlled Voltage Source1/RConn1
  Diode1/LConn1 -- Current Measurement1/RConn1
  -/RConn1 -- Controlled Voltage Source1/LConn1
  Diode1/RConn1 -- +/RConn1

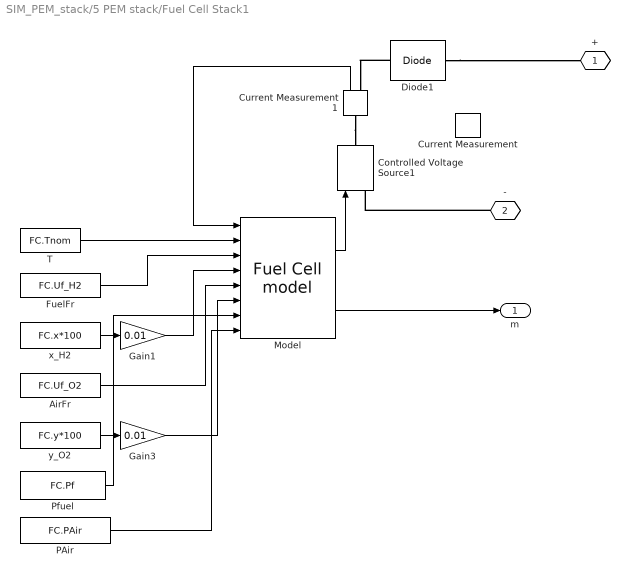
== system SIM_PEM_stack/5 PEM stack/Fuel Cell Stack1 ==
  AirFr : Constant  Value=FC.Uf_O2
  Controlled Voltage Source1 : powerlib/Electrical Sources/Controlled Voltage Source  Initialize=on  Source_Type=AC  Amplitude=0  Phase=0  Frequency=0  Measurements=None
  Current Measurement : powerlib/Measurements/Current Measurement  PhasorSimulation=off  OutputType=Complex  PSBequivalent=0
  Current Measurement1 : powerlib/Measurements/Current Measurement  PhasorSimulation=off  OutputType=Complex  PSBequivalent=0
  Diode1 : powerlib/Power Electronics/Diode  Ron=FC.Rohm  Lon=0  Vf=0  IC=0  UseSnubber=off  Rs=1e4  Cs=inf  Measurements=off
  FuelFr : Constant  Value=FC.Uf_H2
  Gain1 : Gain  Gain=0.01
  Gain3 : Gain  Gain=0.01
  Model : spsFuelCellModel/Fuel Cell model  SystemSampleTime=-1  LabelModeActiveChoice=Continuous/Detailed  VariantActivationTime=update diagram  Latency=0  AutoFrameSizeCalculation=off
      settings: AttributesFormatString=%<BlockChoice>  SourceProductBaseCode=PS
  PAir : Constant  Value=FC.PAir
  Pfuel : Constant  Value=FC.Pf
  T : Constant  Value=FC.Tnom
  x_H2 : Constant  Value=FC.x*100
  y_O2 : Constant  Value=FC.y*100
  + : PMIOPort  Tag=PMCPort  Side=Right
  - : PMIOPort  Tag=PMCPort  Port=2  Side=Right
  m : Outport  VectorParamsAs1DForOutWhenUnconnected=off
  wires:
  PAir/1 -> Model/8
  Pfuel/1 -> Model/7
  T/1 -> Model/2
  Model/1 -> Controlled Voltage Source1/1
  Current Measurement1/1 -> Model/1
  Model/2 -> m/1
  FuelFr/1 -> Model/3
  x_H2/1 -> Gain1/1
  AirFr/1 -> Model/5
  y_O2/1 -> Gain3/1
  Gain1/1 -> Model/4
  Gain3/1 -> Model/6
  connections:
  Current Measurement1/LConn1 -- Controlled Voltage Source1/RConn1
  Diode1/LConn1 -- Current Measurement1/RConn1
  -/RConn1 -- Controlled Voltage Source1/LConn1
  Diode1/RConn1 -- +/RConn1

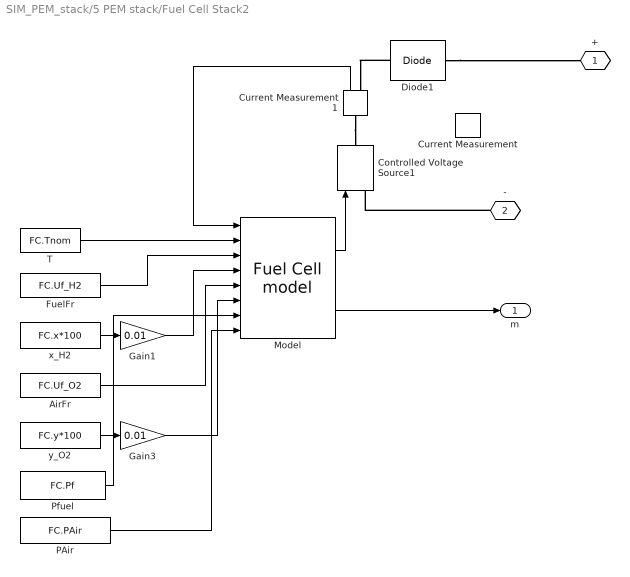
== system SIM_PEM_stack/5 PEM stack/Fuel Cell Stack2 ==
  AirFr : Constant  Value=FC.Uf_O2
  Controlled Voltage Source1 : powerlib/Electrical Sources/Controlled Voltage Source  Initialize=on  Source_Type=AC  Amplitude=0  Phase=0  Frequency=0  Measurements=None
  Current Measurement : powerlib/Measurements/Current Measurement  PhasorSimulation=off  OutputType=Complex  PSBequivalent=0
  Current Measurement1 : powerlib/Measurements/Current Measurement  PhasorSimulation=off  OutputType=Complex  PSBequivalent=0
  Diode1 : powerlib/Power Electronics/Diode  Ron=FC.Rohm  Lon=0  Vf=0  IC=0  UseSnubber=off  Rs=1e4  Cs=inf  Measurements=off
  FuelFr : Constant  Value=FC.Uf_H2
  Gain1 : Gain  Gain=0.01
  Gain3 : Gain  Gain=0.01
  Model : spsFuelCellModel/Fuel Cell model  SystemSampleTime=-1  LabelModeActiveChoice=Continuous/Detailed  VariantActivationTime=update diagram  Latency=0  AutoFrameSizeCalculation=off
      settings: AttributesFormatString=%<BlockChoice>  SourceProductBaseCode=PS
  PAir : Constant  Value=FC.PAir
  Pfuel : Constant  Value=FC.Pf
  T : Constant  Value=FC.Tnom
  x_H2 : Constant  Value=FC.x*100
  y_O2 : Constant  Value=FC.y*100
  + : PMIOPort  Tag=PMCPort  Side=Right
  - : PMIOPort  Tag=PMCPort  Port=2  Side=Right
  m : Outport  VectorParamsAs1DForOutWhenUnconnected=off
  wires:
  PAir/1 -> Model/8
  Pfuel/1 -> Model/7
  T/1 -> Model/2
  Model/1 -> Controlled Voltage Source1/1
  Current Measurement1/1 -> Model/1
  Model/2 -> m/1
  FuelFr/1 -> Model/3
  x_H2/1 -> Gain1/1
  AirFr/1 -> Model/5
  y_O2/1 -> Gain3/1
  Gain1/1 -> Model/4
  Gain3/1 -> Model/6
  connections:
  Current Measurement1/LConn1 -- Controlled Voltage Source1/RConn1
  Diode1/LConn1 -- Current Measurement1/RConn1
  -/RConn1 -- Controlled Voltage Source1/LConn1
  Diode1/RConn1 -- +/RConn1

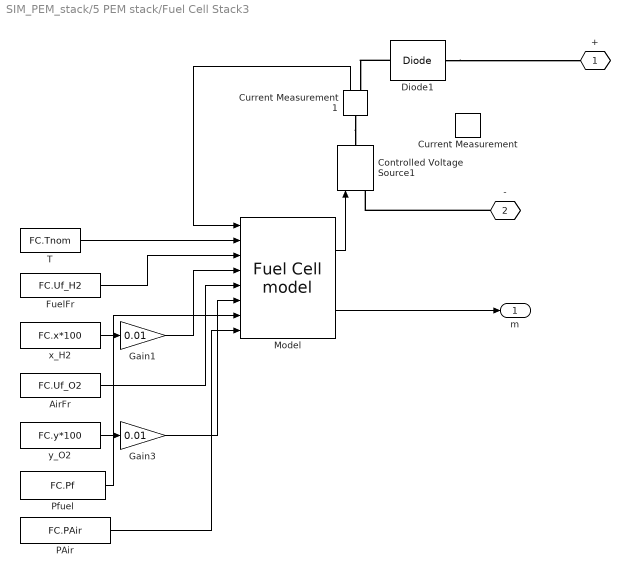
== system SIM_PEM_stack/5 PEM stack/Fuel Cell Stack3 ==
  AirFr : Constant  Value=FC.Uf_O2
  Controlled Voltage Source1 : powerlib/Electrical Sources/Controlled Voltage Source  Initialize=on  Source_Type=AC  Amplitude=0  Phase=0  Frequency=0  Measurements=None
  Current Measurement : powerlib/Measurements/Current Measurement  PhasorSimulation=off  OutputType=Complex  PSBequivalent=0
  Current Measurement1 : powerlib/Measurements/Current Measurement  PhasorSimulation=off  OutputType=Complex  PSBequivalent=0
  Diode1 : powerlib/Power Electronics/Diode  Ron=FC.Rohm  Lon=0  Vf=0  IC=0  UseSnubber=off  Rs=1e4  Cs=inf  Measurements=off
  FuelFr : Constant  Value=FC.Uf_H2
  Gain1 : Gain  Gain=0.01
  Gain3 : Gain  Gain=0.01
  Model : spsFuelCellModel/Fuel Cell model  SystemSampleTime=-1  LabelModeActiveChoice=Continuous/Detailed  VariantActivationTime=update diagram  Latency=0  AutoFrameSizeCalculation=off
      settings: AttributesFormatString=%<BlockChoice>  SourceProductBaseCode=PS
  PAir : Constant  Value=FC.PAir
  Pfuel : Constant  Value=FC.Pf
  T : Constant  Value=FC.Tnom
  x_H2 : Constant  Value=FC.x*100
  y_O2 : Constant  Value=FC.y*100
  + : PMIOPort  Tag=PMCPort  Side=Right
  - : PMIOPort  Tag=PMCPort  Port=2  Side=Right
  m : Outport  VectorParamsAs1DForOutWhenUnconnected=off
  wires:
  PAir/1 -> Model/8
  Pfuel/1 -> Model/7
  T/1 -> Model/2
  Model/1 -> Controlled Voltage Source1/1
  Current Measurement1/1 -> Model/1
  Model/2 -> m/1
  FuelFr/1 -> Model/3
  x_H2/1 -> Gain1/1
  AirFr/1 -> Model/5
  y_O2/1 -> Gain3/1
  Gain1/1 -> Model/4
  Gain3/1 -> Model/6
  connections:
  Current Measurement1/LConn1 -- Controlled Voltage Source1/RConn1
  Diode1/LConn1 -- Current Measurement1/RConn1
  -/RConn1 -- Controlled Voltage Source1/LConn1
  Diode1/RConn1 -- +/RConn1
